simulink library "UAS_Model_library"  (R2018b)
settings: Solver=VariableStepAuto  StartTime=0.0  StopTime=10.0  RelTol=1e-3
undefined symbols (not defined in the file): B, CBAR, CD_alpha, CL_alpha, Cl_beta, Cl_del_a, CL_del_e, Cl_del_r, Cl_p, CL_q, Cl_r, CL_u, Cm_alpha, Cm_alpha_dot, Cm_del_e, Cm_q, Cm_u, Cn_beta, Cn_del_a, Cn_del_r, Cn_p, Cn_r, CY_beta, CY_del_r, CY_p, CY_r, ETA, F, I_TENSOR, Init_Euler, Init_Pos, Init_Rate, Init_Vel, K_p, K_q, K_r, K_roll, K_theta, K_vt, Light, Mass, Max_del_a, Max_del_e, Max_del_r, Max_del_T, MIL, S, tau_a, tau_e, tau_r, tau_T, u_trim, UNIT_GRAV, UNIT_HP2W, XCG, XCGR, XPROP
libraries: aerolibwind2 x3, aerolibasang x3, shared6dofsys x2, aerolibtransform2 x2, aerolibatmos2 x1, sharedtransform x1, sharedutil x1, shared6dof x1, aerolibbdyn x1
settings Model: Creator=e804440  LastModifiedBy=e804440

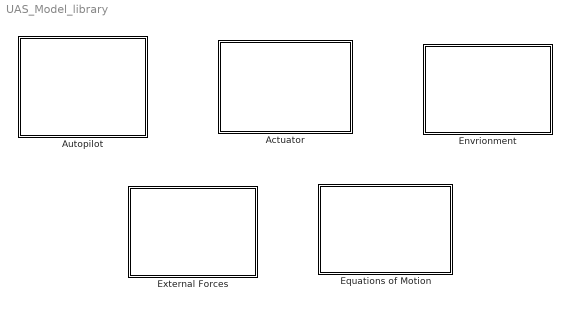
== system UAS_Model_library ==
  Actuator : Subsystem
  Autopilot : Subsystem
  Envrionment : Subsystem
  Equations of Motion : Subsystem
  External Forces : Subsystem

== system UAS_Model_library/Actuator ==
  Aileron Servo : Subsystem
  Elevator Servo : Subsystem
  Rudder Servo : Subsystem
  Throttle Servo : Subsystem

== system UAS_Model_library/Autopilot ==
  Pitch Control : Subsystem
  Roll Control : Subsystem
  Speed Control : Subsystem
  Yaw SAS : Subsystem

== system UAS_Model_library/Envrionment ==
  Atmosphere Model : Subsystem
  Gravity : Subsystem
  Wind Model : Subsystem

== system UAS_Model_library/Equations of Motion ==
  Altitude : Subsystem
  Calculate DCM & Euler Angles : Subsystem
  Calculate omega_dot : shared6dofsys/Calculate omega_dot  aMode=aMode
      settings: SourceProductName=Aerospace Blockset  SourceProductBaseCode=AE
  "Determine Force, Moment & Inertia" : Subsystem
  Vbxw : sharedutil/3x3 Cross Product  aMode=aMode
      settings: SourceProductBaseCode=AE
  "p,q,r " : Integrator  InitialCondition=Init_Rate
  "transform to Inertial axes " : shared6dof/6DOF (Euler Angles)/transform to Inertial axes   SystemSampleTime=-1
      settings: SourceProductName=Aerospace Blockset  SourceProductBaseCode=AE
  ub,vb,wb : Integrator  InitialCondition=Init_Vel
  xe,ye,ze : Integrator  InitialCondition=Init_Pos

== system UAS_Model_library/External Forces ==
  Aerodynamics : Subsystem
  Propulsive : Subsystem
  Total Force & Moment : Subsystem

== system UAS_Model_library/Actuator/Aileron Servo ==
  del_a_cmd : Inport
  Aileron Limit : Saturate  UpperLimit=Max_del_a  LowerLimit=-Max_del_a
  Aileron Servo : TransferFcn  Denominator=[tau_a 1]
  Sum2 : Sum  SaturateOnIntegerOverflow=on
  Trim del_T2 : Constant  Value=u_trim(3)
  del_a : Outport
  wires:
  Trim del_T2/1 -> Sum2/2
  Sum2/1 -> Aileron Limit/1
  del_a_cmd/1 -> Aileron Servo/1
  Aileron Servo/1 -> Sum2/1
  Aileron Limit/1 -> del_a/1

== system UAS_Model_library/Actuator/Elevator Servo ==
  del_e_cmd : Inport
  Elevator Limit : Saturate  UpperLimit=Max_del_e  LowerLimit=-Max_del_e
  Elevator Servo : TransferFcn  Numerator=[-1]  Denominator=[tau_e 1]
  Sum1 : Sum  SaturateOnIntegerOverflow=on
  Trim del_T1 : Constant  Value=u_trim(2)
  del_e : Outport
  wires:
  Sum1/1 -> Elevator Limit/1
  del_e_cmd/1 -> Elevator Servo/1
  Trim del_T1/1 -> Sum1/2
  Elevator Servo/1 -> Sum1/1
  Elevator Limit/1 -> del_e/1

== system UAS_Model_library/Actuator/Rudder Servo ==
  del_r_cmd : Inport
  Rudder Limit : Saturate  UpperLimit=Max_del_r  LowerLimit=-Max_del_r
  Rudder Servo : TransferFcn  Numerator=[-1]  Denominator=[tau_r 1]
  Sum3 : Sum  SaturateOnIntegerOverflow=on
  Trim del_T3 : Constant  Value=u_trim(4)
  del_r : Outport
  wires:
  Trim del_T3/1 -> Sum3/2
  Rudder Limit/1 -> del_r/1
  Rudder Servo/1 -> Sum3/1
  del_r_cmd/1 -> Rudder Servo/1
  Sum3/1 -> Rudder Limit/1

== system UAS_Model_library/Actuator/Throttle Servo ==
  del_T_cmd : Inport
  Sum : Sum  SaturateOnIntegerOverflow=on
  Throttle Limit : Saturate  UpperLimit=Max_del_T  LowerLimit=-Max_del_T
  Throttle Servo : TransferFcn  Denominator=[tau_T 1]
  Trim del_T : Constant  Value=u_trim(1)
  del_T : Outport
  wires:
  del_T_cmd/1 -> Throttle Servo/1
  Sum/1 -> Throttle Limit/1
  Throttle Servo/1 -> Sum/1
  Trim del_T/1 -> Sum/2
  Throttle Limit/1 -> del_T/1

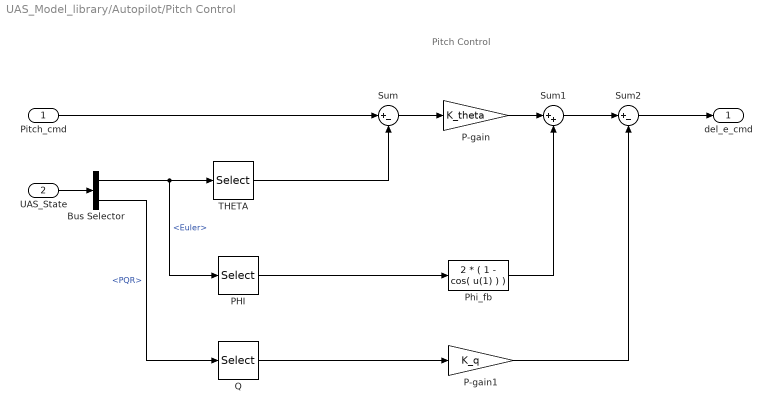
== system UAS_Model_library/Autopilot/Pitch Control ==
  note: Pitch Control
  Pitch_cmd : Inport
  UAS_State : Inport  Port=2
  Bus Selector : BusSelector  OutputSignals=Euler,PQR
  P-gain : Gain  Gain=K_theta
  P-gain1 : Gain  Gain=K_q
  PHI : Selector  InputPortWidth=3  IndexOptions=Index vector (dialog)  Indices=[1]  OutputSizes=1
  Phi_fb : Fcn  Expr=2 * ( 1 - cos( u(1) ) )
  Q : Selector  InputPortWidth=3  IndexOptions=Index vector (dialog)  Indices=[2]  OutputSizes=1
  Sum : Sum  Inputs=|+-
  Sum1 : Sum  Inputs=|++
  Sum2 : Sum  Inputs=|+-
  THETA : Selector  InputPortWidth=3  IndexOptions=Index vector (dialog)  Indices=[2]  OutputSizes=1
  del_e_cmd : Outport
  wires:
  Pitch_cmd/1 -> Sum/1
  Sum/1 -> P-gain/1
  THETA/1 -> Sum/2
  P-gain/1 -> Sum1/1
  Q/1 -> P-gain1/1
  PHI/1 -> Phi_fb/1
  Phi_fb/1 -> Sum1/2
  Sum1/1 -> Sum2/1
  P-gain1/1 -> Sum2/2
  Sum2/1 -> del_e_cmd/1
  Bus Selector/1 -> PHI/1, THETA/1  "<Euler>"
  UAS_State/1 -> Bus Selector/1
  Bus Selector/2 -> Q/1  "<PQR>"

== system UAS_Model_library/Autopilot/Roll Control ==
  note: Roll Control
  Roll_cmd : Inport
  UAS_State : Inport  Port=2
  Bus Selector : BusSelector  OutputSignals=Euler,PQR
  Discrete Transfer Fcn : DiscreteTransferFcn  Numerator=[K_roll -K_roll]  Denominator=[1 -1]
  P : Selector  InputPortWidth=3  IndexOptions=Index vector (dialog)  Indices=[1]  OutputSizes=1
  P-gain1 : Gain  Gain=K_p
  PHI : Selector  InputPortWidth=3  IndexOptions=Index vector (dialog)  Indices=[1]  OutputSizes=1
  Sum : Sum  Inputs=|+-
  Sum2 : Sum  Inputs=|+-
  del_a_cmd : Outport
  wires:
  Sum2/1 -> del_a_cmd/1
  P-gain1/1 -> Sum2/2
  Discrete Transfer Fcn/1 -> Sum2/1
  P/1 -> P-gain1/1
  Sum/1 -> Discrete Transfer Fcn/1
  Roll_cmd/1 -> Sum/1
  PHI/1 -> Sum/2
  UAS_State/1 -> Bus Selector/1
  Bus Selector/1 -> PHI/1  "<Euler>"
  Bus Selector/2 -> P/1  "<PQR>"

== system UAS_Model_library/Autopilot/Speed Control ==
  note: Speed Control
  Speed_cmd : Inport
  UAS_State : Inport  Port=2
  Bus Selector : BusSelector  OutputSignals=Alpha_Beta_V
  P-gain : Gain  Gain=K_vt
  Sum : Sum  Inputs=|+-
  VT : Selector  InputPortWidth=3  IndexOptions=Index vector (dialog)  Indices=[3]  OutputSizes=1
  del_T_cmd : Outport
  wires:
  P-gain/1 -> del_T_cmd/1
  UAS_State/1 -> Bus Selector/1
  VT/1 -> Sum/2
  Sum/1 -> P-gain/1
  Speed_cmd/1 -> Sum/1
  Bus Selector/1 -> VT/1  "<Alpha_Beta_V>"

== system UAS_Model_library/Autopilot/Yaw SAS ==
  note: Yaw SAS (Stability Augmented System)
  UAS_State : Inport
  Bus Selector : BusSelector  OutputSignals=PQR
  P-gain1 : Gain  Gain=K_r
  R : Selector  InputPortWidth=3  IndexOptions=Index vector (dialog)  Indices=[3]  OutputSizes=1
  del_r_cmd : Outport
  wires:
  UAS_State/1 -> Bus Selector/1
  R/1 -> P-gain1/1
  P-gain1/1 -> del_r_cmd/1
  Bus Selector/1 -> R/1  "<PQR>"

== system UAS_Model_library/Envrionment/Atmosphere Model ==
  Alt : Inport
  ISA Atmosphere Model : aerolibatmos2/ISA Atmosphere Model  custom=off  g=9.80665  gamma=1.4  R=287.0531  L=0.0065  h_trop=11000  h_strat=20000  rho0=1.225  P0=101325  T0=288.15  h0=0
      settings: SourceProductName=Aerospace Blockset
  Terminator : Terminator
  Terminator1 : Terminator
  a : Outport
  rho : Outport  Port=2
  wires:
  ISA Atmosphere Model/3 -> Terminator1/1
  ISA Atmosphere Model/1 -> Terminator/1
  ISA Atmosphere Model/4 -> rho/1
  Alt/1 -> ISA Atmosphere Model/1
  ISA Atmosphere Model/2 -> a/1

== system UAS_Model_library/Envrionment/Gravity ==
  cE_B : Inport
  Constant : Constant  Value=0
  Constant1 : Constant  Value=Mass
  "Gravity vector in body frame " : Product  Multiplication=Matrix(*)  SaturateOnIntegerOverflow=on  InputSameDT=on  OutDataTypeStr=Inherit: Same as first input
  Mux1 : Mux  Inputs=3
  g : Gain  Gain=UNIT_GRAV
  Gravity : Outport
  wires:
  Constant/1 -> Mux1/2, Mux1/1
  cE_B/1 -> "Gravity vector in body frame "/1
  Mux1/1 -> "Gravity vector in body frame "/2
  g/1 -> Mux1/3
  "Gravity vector in body frame "/1 -> Gravity/1
  Constant1/1 -> g/1

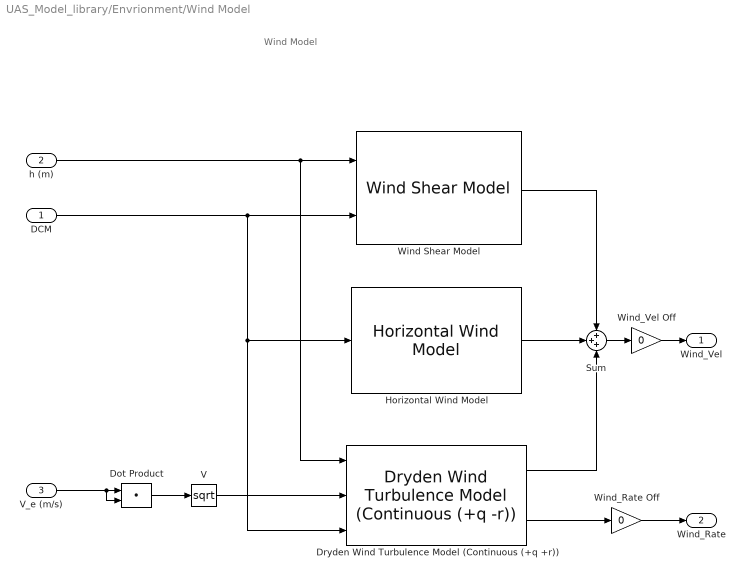
== system UAS_Model_library/Envrionment/Wind Model ==
  note: Wind Model
  DCM : Inport
  h (m) : Inport  Port=2
  V_e (m/s) : Inport  Port=3
  Dot Product : DotProduct  SaturateOnIntegerOverflow=on  OutDataTypeStr=Inherit: Inherit via internal rule
  Dryden Wind Turbulence Model (Continuous (+q +r)) : aerolibwind2/Dryden Wind Turbulence Model  (Continuous (+q -r))  units=Metric (MKS)  spec=MIL-F-8785C  model=Continuous Dryden (+q -r)  W20=15  Wdeg=0  TurbProb=10^-2 - Light  L_high=533.4  Wingspan=B  ts=Step_Size  Seed=[23341 23342 23343 23344]  T_on=off
      settings: SourceProductName=Aerospace Blockset
  Horizontal Wind Model : aerolibwind2/Horizontal Wind Model  units=Metric (MKS)  Vw_source=Internal  Vwind=0  W_source=Internal  Wdeg=0
      settings: SourceProductName=Aerospace Blockset  SourceProductBaseCode=AE
  Sum : Sum  Inputs=+++  SaturateOnIntegerOverflow=on  InputSameDT=on  OutDataTypeStr=Inherit: Same as first input
  V : Math  Operator=sqrt  SaturateOnIntegerOverflow=on
  Wind Shear Model : aerolibwind2/Wind Shear Model  units=Metric (MKS)  phase=Category C - Terminal Flight Phase  W_20=0  Wdeg=0
      settings: SourceProductName=Aerospace Blockset
  Wind_Rate Off : Gain  Gain=0
  Wind_Vel Off : Gain  Gain=0
  Wind_Vel : Outport
  Wind_Rate : Outport  Port=2
  wires:
  Wind_Rate Off/1 -> Wind_Rate/1
  Wind_Vel Off/1 -> Wind_Vel/1
  V/1 -> Dryden Wind Turbulence Model (Continuous (+q +r))/2
  DCM/1 -> Wind Shear Model/2, Horizontal Wind Model/1, Dryden Wind Turbulence Model (Continuous (+q +r))/3
  h (m)/1 -> Wind Shear Model/1, Dryden Wind Turbulence Model (Continuous (+q +r))/1
  Dryden Wind Turbulence Model (Continuous (+q +r))/1 -> Sum/3
  V_e (m/s)/1 -> Dot Product/1, Dot Product/2
  Dot Product/1 -> V/1
  Dryden Wind Turbulence Model (Continuous (+q +r))/2 -> Wind_Rate Off/1
  Sum/1 -> Wind_Vel Off/1
  Horizontal Wind Model/1 -> Sum/2
  Wind Shear Model/1 -> Sum/1

== system UAS_Model_library/Equations of Motion/Altitude ==
  Xe : Inport
  Z_e : Selector  InputPortWidth=3  IndexOptions=Index vector (dialog)  Indices=[3]  OutputSizes=1
  conv : Gain  Gain=-1
  h : Outport
  wires:
  conv/1 -> h/1
  Z_e/1 -> conv/1
  Xe/1 -> Z_e/1

== system UAS_Model_library/Equations of Motion/Calculate DCM & Euler Angles ==
  "p q r " : Inport
  Rotation Angles to Direction Cosine Matrix : sharedtransform/Rotation Angles to Direction Cosine Matrix  rotationOrder=ZYX  aMode=aMode
      settings: SourceProductBaseCode=AE
  Selector : Selector  InputPortWidth=3  IndexOptions=Index vector (dialog)  Indices=[3 2 1]  OutputSizes=1
  phi theta psi : Integrator  InitialCondition=Init_Euler
  phidot thetadot psidot : shared6dofsys/DCM & Euler Angles (Euler)/phidot thetadot psidot  SystemSampleTime=-1
      settings: SourceProductName=Aerospace Blockset  SourceProductBaseCode=AE
  DCM : Outport
  Euler : Outport  Port=2
  wires:
  Selector/1 -> Rotation Angles to Direction Cosine Matrix/1
  phi theta psi/1 -> phidot thetadot psidot/2, Selector/1, Euler/1
  phidot thetadot psidot/1 -> phi theta psi/1
  "p q r "/1 -> phidot thetadot psidot/1
  Rotation Angles to Direction Cosine Matrix/1 -> DCM/1

== system UAS_Model_library/Equations of Motion/Determine Force, Moment & Inertia ==
  forces : Inport
  Constant : Constant  Value=Mass  OutDataTypeStr=Inherit: Inherit via back propagation
  Constant1 : Constant  Value=I_TENSOR  OutDataTypeStr=Inherit: Inherit via back propagation
  Constant2 : Constant  Value=zeros(3)
  Vector Concatenate : Concatenate  Mode=Multidimensional array
  "forces " : Outport
  mass : Outport  Port=2
  "inertia, 0" : Outport  Port=3
  wires:
  Vector Concatenate/1 -> "inertia, 0"/1
  Constant2/1 -> Vector Concatenate/2
  Constant1/1 -> Vector Concatenate/1
  forces/1 -> "forces "/1
  Constant/1 -> mass/1

== system UAS_Model_library/External Forces/Aerodynamics ==
  Aerodynamic Force & Moment : Subsystem
  Aerodynamics coefficients : Subsystem
  Direction Cosine Matrix Body to Wind : aerolibtransform2/Direction Cosine Matrix Body to Wind
      settings: SourceProductName=Aerospace Blockset  SourceProductBaseCode=AE
  Wind-axes Velocitie : Subsystem

== system UAS_Model_library/External Forces/Propulsive ==
  Propulsive Force & Moment : Subsystem

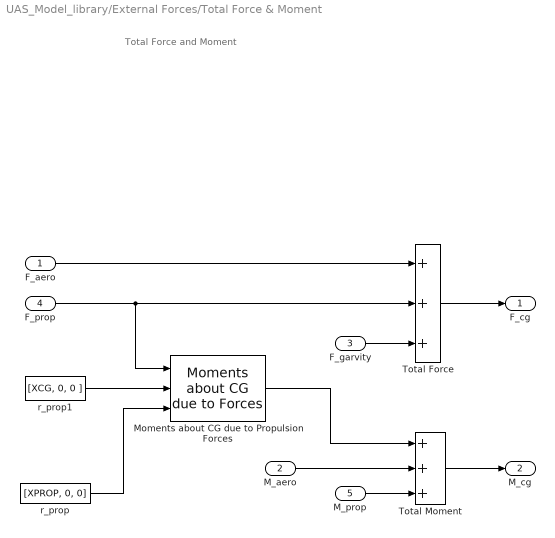
== system UAS_Model_library/External Forces/Total Force & Moment ==
  note: Total Force and Moment
  F_aero : Inport  PortDimensions=3
  M_aero : Inport  Port=2  PortDimensions=3
  F_garvity : Inport  Port=3  PortDimensions=3
  F_prop : Inport  Port=4  PortDimensions=3
  M_prop : Inport  Port=5  PortDimensions=3
  Moments about CG due to Propulsion Forces : aerolibbdyn/Moments about CG  due to Forces
      settings: SourceProductName=Aerospace Blockset  SourceProductBaseCode=AE
  Total Force : Sum  Inputs=+++  SaturateOnIntegerOverflow=on  InputSameDT=on  OutDataTypeStr=Inherit: Same as first input
  Total Moment : Sum  Inputs=+++  SaturateOnIntegerOverflow=on  InputSameDT=on  OutDataTypeStr=Inherit: Same as first input
  r_prop : Constant  Value=[XPROP, 0, 0]  OutDataTypeStr=double
  r_prop1 : Constant  Value=[XCG, 0, 0 ]  OutDataTypeStr=double
  F_cg : Outport
  M_cg : Outport  Port=2
  wires:
  M_aero/1 -> Total Moment/2
  Moments about CG due to Propulsion Forces/1 -> Total Moment/1
  Total Force/1 -> F_cg/1
  F_aero/1 -> Total Force/1
  F_prop/1 -> Moments about CG due to Propulsion Forces/1, Total Force/2
  M_prop/1 -> Total Moment/3
  Total Moment/1 -> M_cg/1
  r_prop/1 -> Moments about CG due to Propulsion Forces/3
  r_prop1/1 -> Moments about CG due to Propulsion Forces/2
  F_garvity/1 -> Total Force/3

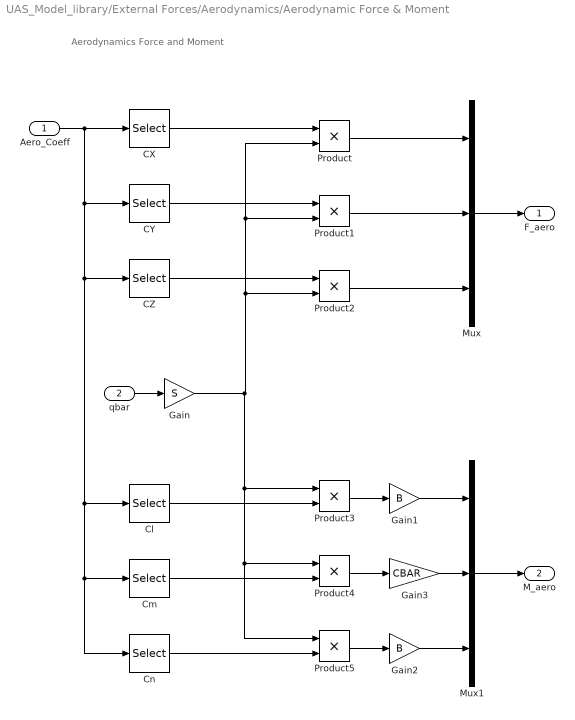
== system UAS_Model_library/External Forces/Aerodynamics/Aerodynamic Force & Moment ==
  note: Aerodynamics Force and Moment
  Aero_Coeff : Inport
  qbar : Inport  Port=2
  CX : Selector  InputPortWidth=6  IndexOptions=Index vector (dialog)  Indices=[1]  OutputSizes=1
  CY : Selector  InputPortWidth=6  IndexOptions=Index vector (dialog)  Indices=[2]  OutputSizes=1
  CZ : Selector  InputPortWidth=6  IndexOptions=Index vector (dialog)  Indices=[3]  OutputSizes=1
  Cl : Selector  InputPortWidth=6  IndexOptions=Index vector (dialog)  Indices=[4]  OutputSizes=1
  Cm : Selector  InputPortWidth=6  IndexOptions=Index vector (dialog)  Indices=[5]  OutputSizes=1
  Cn : Selector  InputPortWidth=6  IndexOptions=Index vector (dialog)  Indices=[6]  OutputSizes=1
  Gain : Gain  Gain=S
  Gain1 : Gain  Gain=B
  Gain2 : Gain  Gain=B
  Gain3 : Gain  Gain=CBAR
  Mux : Mux  Inputs=3
  Mux1 : Mux  Inputs=3
  Product{,1..5} (6 alike) : Product
  F_aero : Outport
  M_aero : Outport  Port=2
  wires:
  Aero_Coeff/1 -> Cl/1, Cn/1, Cm/1, CZ/1, CY/1, CX/1
  qbar/1 -> Gain/1
  CX/1 -> Product/1
  Gain/1 -> Product5/1, Product4/1, Product3/1, Product2/2, Product1/2, Product/2
  CY/1 -> Product1/1
  CZ/1 -> Product2/1
  Product/1 -> Mux/1
  Product1/1 -> Mux/2
  Product2/1 -> Mux/3
  Mux/1 -> F_aero/1
  Cl/1 -> Product3/2
  Cm/1 -> Product4/2
  Cn/1 -> Product5/2
  Product3/1 -> Gain1/1
  Product4/1 -> Gain3/1
  Product5/1 -> Gain2/1
  Mux1/1 -> M_aero/1
  Gain1/1 -> Mux1/1
  Gain2/1 -> Mux1/3
  Gain3/1 -> Mux1/2

== system UAS_Model_library/External Forces/Aerodynamics/Aerodynamics coefficients ==
  Drag Force Coefficient : Subsystem
  "Lift Force Coefficient  " : Subsystem
  Pitching Moment Coefficient : Subsystem
  Rolling Moment Coefficient : Subsystem
  "Side Force Coefficient " : Subsystem
  Yawing Moment Coefficient : Subsystem

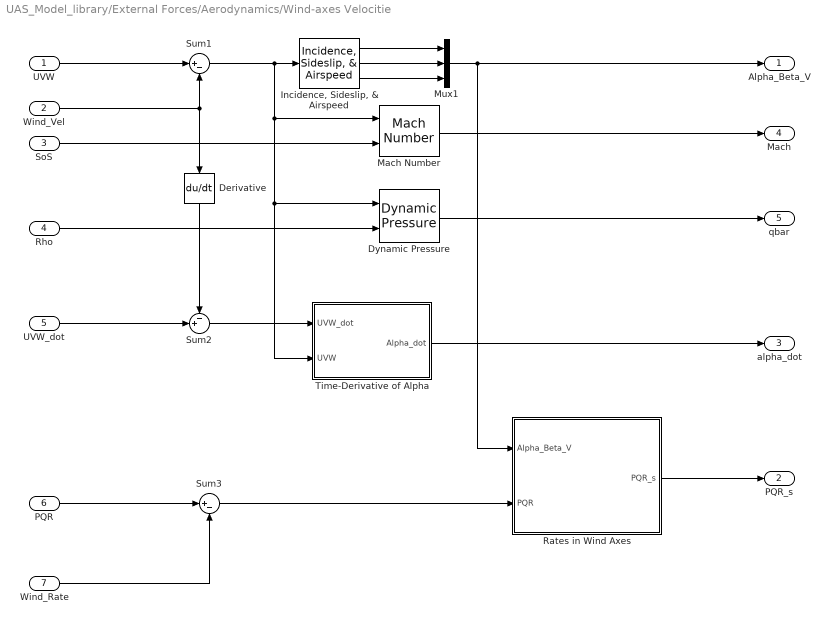
== system UAS_Model_library/External Forces/Aerodynamics/Wind-axes Velocitie ==
  UVW : Inport
  Wind_Vel : Inport  Port=2
  SoS : Inport  Port=3
  Rho : Inport  Port=4
  UVW_dot : Inport  Port=5
  PQR : Inport  Port=6
  Wind_Rate : Inport  Port=7
  Derivative : Derivative
  Dynamic Pressure : aerolibasang/Dynamic Pressure
  "Incidence, Sideslip, & Airspeed" : aerolibasang/Incidence, Sideslip, & Airspeed
      settings: SourceProductName=Aerospace Blockset
  Mach Number : aerolibasang/Mach Number
      settings: SourceProductName=Aerospace Blockset  SourceProductBaseCode=AE
  Mux1 : Mux  Inputs=3
  Rates in Wind Axes : Subsystem
  Sum1 : Sum  Inputs=|+-  SaturateOnIntegerOverflow=on  InputSameDT=on  OutDataTypeStr=Inherit: Same as first input
  Sum2 : Sum  Inputs=-+|  SaturateOnIntegerOverflow=on  InputSameDT=on  OutDataTypeStr=Inherit: Same as first input
  Sum3 : Sum  Inputs=|+-  SaturateOnIntegerOverflow=on  InputSameDT=on  OutDataTypeStr=Inherit: Same as first input
  Time-Derivative of Alpha : Subsystem
  Alpha_Beta_V : Outport
  PQR_s : Outport  Port=2
  alpha_dot : Outport  Port=3
  Mach : Outport  Port=4
  qbar : Outport  Port=5
  wires:
  Derivative/1 -> Sum2/1
  Sum2/1 -> Time-Derivative of Alpha/1(UVW_dot)
  UVW_dot/1 -> Sum2/2
  Time-Derivative of Alpha/1(Alpha_dot) -> alpha_dot/1
  Dynamic Pressure/1 -> qbar/1
  Rho/1 -> Dynamic Pressure/2
  SoS/1 -> Mach Number/2
  Mach Number/1 -> Mach/1
  Wind_Vel/1 -> Sum1/2, Derivative/1
  UVW/1 -> Sum1/1
  Mux1/1 -> Rates in Wind Axes/1(Alpha_Beta_V), Alpha_Beta_V/1
  Sum1/1 -> Time-Derivative of Alpha/2(UVW), Dynamic Pressure/1, Mach Number/1, "Incidence, Sideslip, & Airspeed"/1
  "Incidence, Sideslip, & Airspeed"/1 -> Mux1/1
  "Incidence, Sideslip, & Airspeed"/2 -> Mux1/2
  "Incidence, Sideslip, & Airspeed"/3 -> Mux1/3
  Rates in Wind Axes/1(PQR_s) -> PQR_s/1
  Sum3/1 -> Rates in Wind Axes/2(PQR)
  PQR/1 -> Sum3/1
  Wind_Rate/1 -> Sum3/2

== system UAS_Model_library/External Forces/Propulsive/Propulsive Force & Moment ==
  note: Propulsive Force and Moment
  Controls : Inport
  Alpha_Beta_V : Inport  Port=2
  Constant : Constant  Value=0
  Engine Thrust : Product  Inputs=*/
  Gain : Gain  Gain=ETA
  Gain1 : Gain  Gain=UNIT_HP2W
  Mux : Mux  Inputs=3
  Mux1 : Mux  Inputs=3
  V : Selector  InputPortWidth=3  IndexOptions=Index vector (dialog)  Indices=[3]  OutputSizes=1
  del_T (HP) : Selector  InputPortWidth=4  IndexOptions=Index vector (dialog)  Indices=[1]  OutputSizes=1
  F_prop : Outport
  M_prop : Outport  Port=2
  wires:
  Mux1/1 -> M_prop/1
  Constant/1 -> Mux/3, Mux1/3, Mux1/2, Mux1/1, Mux/2
  Controls/1 -> del_T (HP)/1
  del_T (HP)/1 -> Gain1/1
  Gain1/1 -> Gain/1
  Gain/1 -> Engine Thrust/1  "Engine Power"
  Engine Thrust/1 -> Mux/1
  Alpha_Beta_V/1 -> V/1
  V/1 -> Engine Thrust/2
  Mux/1 -> F_prop/1

== system UAS_Model_library/External Forces/Aerodynamics/Aerodynamics coefficients/Drag Force Coefficient ==
  note: Drag Force Coefficient
  Alpha_Beta_V : Inport
  Alpha : Selector  InputPortWidth=3  IndexOptions=Index vector (dialog)  Indices=[1]  OutputSizes=1
  Gain : Gain  Gain=CD_alpha
  CD : Outport
  wires:
  Alpha_Beta_V/1 -> Alpha/1
  Alpha/1 -> Gain/1
  Gain/1 -> CD/1

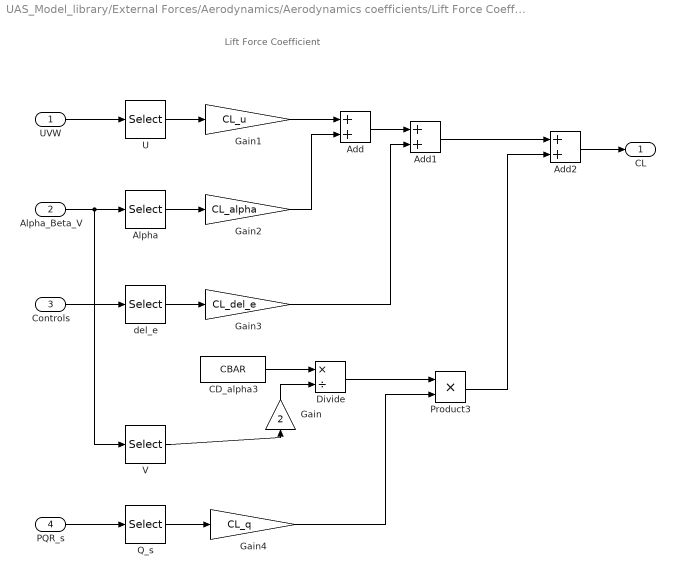
== system UAS_Model_library/External Forces/Aerodynamics/Aerodynamics coefficients/Lift Force Coefficient   ==
  note: Lift Force Coefficient
  UVW : Inport
  Alpha_Beta_V : Inport  Port=2
  Controls : Inport  Port=3
  PQR_s : Inport  Port=4
  Add : Sum
  Add1 : Sum
  Add2 : Sum
  Alpha : Selector  InputPortWidth=3  IndexOptions=Index vector (dialog)  Indices=[1]  OutputSizes=1
  CD_alpha3 : Constant  Value=CBAR
  Divide : Product  Inputs=*/
  Gain : Gain  Gain=2
  Gain1 : Gain  Gain=CL_u
  Gain2 : Gain  Gain=CL_alpha
  Gain3 : Gain  Gain=CL_del_e
  Gain4 : Gain  Gain=CL_q
  Product3 : Product
  Q_s : Selector  InputPortWidth=3  IndexOptions=Index vector (dialog)  Indices=[2]  OutputSizes=1
  U : Selector  InputPortWidth=3  IndexOptions=Index vector (dialog)  Indices=[1]  OutputSizes=1
  V : Selector  InputPortWidth=3  IndexOptions=Index vector (dialog)  Indices=[3]  OutputSizes=1
  del_e : Selector  InputPortWidth=4  IndexOptions=Index vector (dialog)  Indices=[2]  OutputSizes=1
  CL : Outport
  wires:
  UVW/1 -> U/1
  Alpha_Beta_V/1 -> Alpha/1, V/1
  Gain2/1 -> Add/2
  Controls/1 -> del_e/1
  Add/1 -> Add1/1
  Gain3/1 -> Add1/2
  CD_alpha3/1 -> Divide/1
  Gain/1 -> Divide/2
  Divide/1 -> Product3/1
  Add1/1 -> Add2/1
  Product3/1 -> Add2/2
  Add2/1 -> CL/1
  Gain4/1 -> Product3/2
  PQR_s/1 -> Q_s/1
  U/1 -> Gain1/1
  Alpha/1 -> Gain2/1
  del_e/1 -> Gain3/1
  V/1 -> Gain/1
  Q_s/1 -> Gain4/1
  Gain1/1 -> Add/1

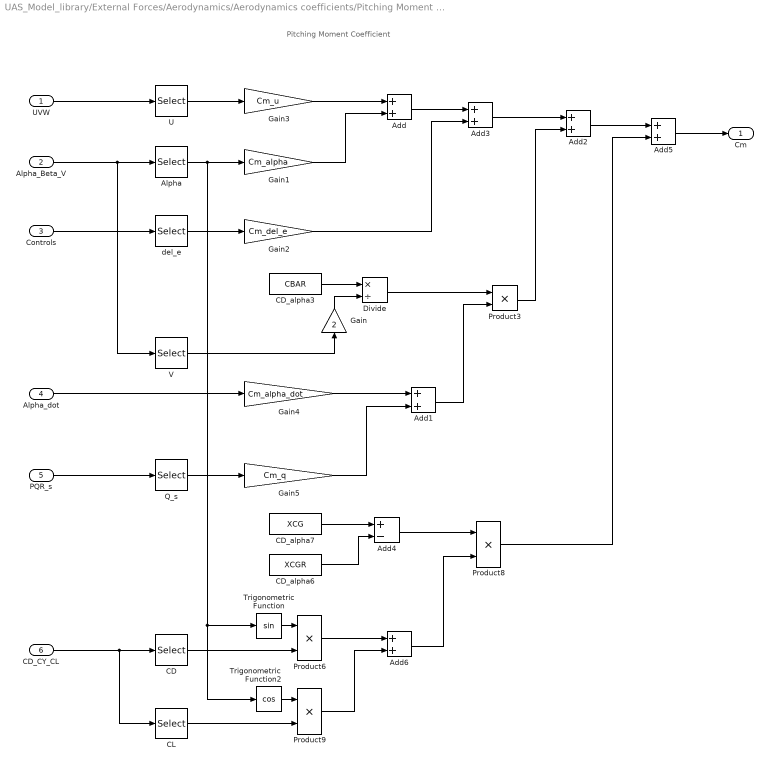
== system UAS_Model_library/External Forces/Aerodynamics/Aerodynamics coefficients/Pitching Moment Coefficient ==
  note: Pitching Moment Coefficient
  UVW : Inport
  Alpha_Beta_V : Inport  Port=2
  Controls : Inport  Port=3
  Alpha_dot : Inport  Port=4
  PQR_s : Inport  Port=5
  CD_CY_CL : Inport  Port=6
  Add{,1..3,5..6} (6 alike) : Sum
  Add4 : Sum  Inputs=+-
  Alpha : Selector  InputPortWidth=3  IndexOptions=Index vector (dialog)  Indices=[1]  OutputSizes=1
  CD : Selector  InputPortWidth=3  IndexOptions=Index vector (dialog)  Indices=[1]  OutputSizes=1
  CD_alpha3 : Constant  Value=CBAR
  CD_alpha6 : Constant  Value=XCGR
  CD_alpha7 : Constant  Value=XCG
  CL : Selector  InputPortWidth=3  IndexOptions=Index vector (dialog)  Indices=[3]  OutputSizes=1
  Divide : Product  Inputs=*/
  Gain : Gain  Gain=2
  Gain1 : Gain  Gain=Cm_alpha
  Gain2 : Gain  Gain=Cm_del_e
  Gain3 : Gain  Gain=Cm_u
  Gain4 : Gain  Gain=Cm_alpha_dot
  Gain5 : Gain  Gain=Cm_q
  Product{3,6,8..9} (4 alike) : Product
  Q_s : Selector  InputPortWidth=3  IndexOptions=Index vector (dialog)  Indices=[2]  OutputSizes=1
  Trigonometric Function : Trigonometry
  Trigonometric Function2 : Trigonometry  Operator=cos
  U : Selector  InputPortWidth=3  IndexOptions=Index vector (dialog)  Indices=[1]  OutputSizes=1
  V : Selector  InputPortWidth=3  IndexOptions=Index vector (dialog)  Indices=[3]  OutputSizes=1
  del_e : Selector  InputPortWidth=4  IndexOptions=Index vector (dialog)  Indices=[2]  OutputSizes=1
  Cm : Outport
  wires:
  UVW/1 -> U/1
  Gain3/1 -> Add/1
  Alpha_Beta_V/1 -> V/1, Alpha/1
  Gain1/1 -> Add/2
  CD_alpha3/1 -> Divide/1
  Gain/1 -> Divide/2
  Divide/1 -> Product3/1
  Add/1 -> Add3/1
  Alpha_dot/1 -> Gain4/1
  PQR_s/1 -> Q_s/1
  Product3/1 -> Add2/2
  Controls/1 -> del_e/1
  Gain2/1 -> Add3/2
  Add3/1 -> Add2/1
  CD_CY_CL/1 -> CL/1, CD/1
  Trigonometric Function/1 -> Product6/1
  CD_alpha7/1 -> Add4/1
  CD_alpha6/1 -> Add4/2
  Add4/1 -> Product8/1
  Product8/1 -> Add5/2
  Add2/1 -> Add5/1
  Add5/1 -> Cm/1
  Gain5/1 -> Add1/2
  Add1/1 -> Product3/2
  Product6/1 -> Add6/1
  Trigonometric Function2/1 -> Product9/1
  Product9/1 -> Add6/2
  Add6/1 -> Product8/2
  U/1 -> Gain3/1
  Alpha/1 -> Gain1/1, Trigonometric Function/1, Trigonometric Function2/1
  del_e/1 -> Gain2/1
  V/1 -> Gain/1
  Q_s/1 -> Gain5/1
  CD/1 -> Product6/2
  CL/1 -> Product9/2
  Gain4/1 -> Add1/1

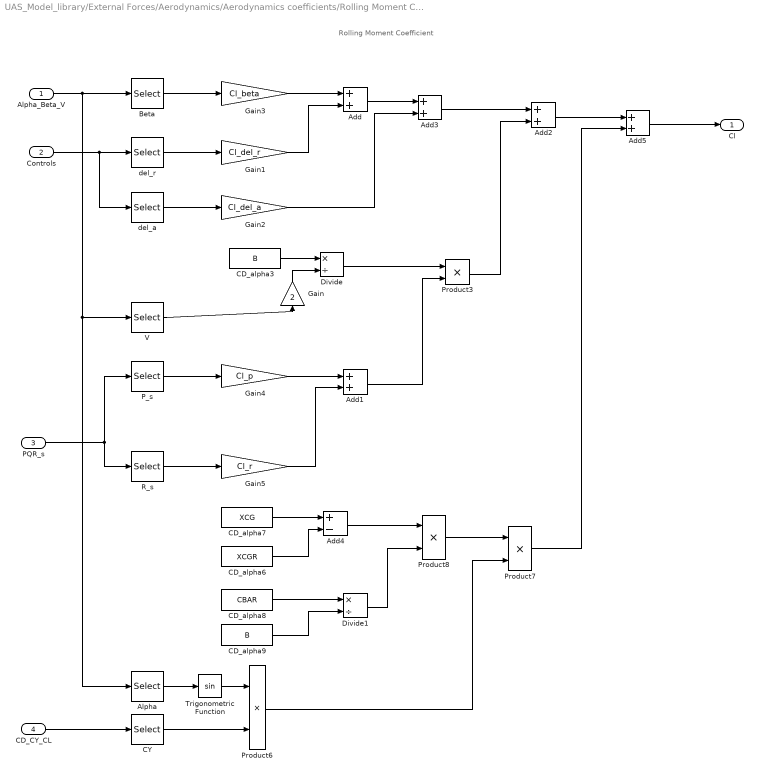
== system UAS_Model_library/External Forces/Aerodynamics/Aerodynamics coefficients/Rolling Moment Coefficient ==
  note: Rolling Moment Coefficient
  Alpha_Beta_V : Inport
  Controls : Inport  Port=2
  PQR_s : Inport  Port=3
  CD_CY_CL : Inport  Port=4
  Add{,1..3,5} (5 alike) : Sum
  Add4 : Sum  Inputs=+-
  Alpha : Selector  InputPortWidth=3  IndexOptions=Index vector (dialog)  Indices=[1]  OutputSizes=1
  Beta : Selector  InputPortWidth=3  IndexOptions=Index vector (dialog)  Indices=[2]  OutputSizes=1
  CD_alpha3 : Constant  Value=B
  CD_alpha6 : Constant  Value=XCGR
  CD_alpha7 : Constant  Value=XCG
  CD_alpha8 : Constant  Value=CBAR
  CD_alpha9 : Constant  Value=B
  CY : Selector  InputPortWidth=3  IndexOptions=Index vector (dialog)  Indices=[2]  OutputSizes=1
  Divide : Product  Inputs=*/
  Divide1 : Product  Inputs=*/
  Gain : Gain  Gain=2
  Gain1 : Gain  Gain=Cl_del_r
  Gain2 : Gain  Gain=Cl_del_a
  Gain3 : Gain  Gain=Cl_beta
  Gain4 : Gain  Gain=Cl_p
  Gain5 : Gain  Gain=Cl_r
  P_s : Selector  InputPortWidth=3  IndexOptions=Index vector (dialog)  Indices=[1]  OutputSizes=1
  Product{3,6..8} (4 alike) : Product
  R_s : Selector  InputPortWidth=3  IndexOptions=Index vector (dialog)  Indices=[3]  OutputSizes=1
  Trigonometric Function : Trigonometry
  V : Selector  InputPortWidth=3  IndexOptions=Index vector (dialog)  Indices=[3]  OutputSizes=1
  del_a : Selector  InputPortWidth=4  IndexOptions=Index vector (dialog)  Indices=[3]  OutputSizes=1
  del_r : Selector  InputPortWidth=4  IndexOptions=Index vector (dialog)  Indices=[4]  OutputSizes=1
  Cl : Outport
  wires:
  Alpha_Beta_V/1 -> Alpha/1, V/1, Beta/1
  Gain3/1 -> Add/1
  Controls/1 -> del_a/1, del_r/1
  Gain1/1 -> Add/2
  CD_alpha3/1 -> Divide/1
  Gain/1 -> Divide/2
  Divide/1 -> Product3/1
  Add/1 -> Add3/1
  Gain4/1 -> Add1/1
  Gain5/1 -> Add1/2
  Add1/1 -> Product3/2
  Product3/1 -> Add2/2
  Add3/1 -> Add2/1
  Trigonometric Function/1 -> Product6/1
  Product6/1 -> Product7/2
  CD_alpha7/1 -> Add4/1
  CD_alpha6/1 -> Add4/2
  Add4/1 -> Product8/1
  Divide1/1 -> Product8/2
  CD_alpha8/1 -> Divide1/1
  CD_alpha9/1 -> Divide1/2
  Product8/1 -> Product7/1
  Add2/1 -> Add5/1
  Add5/1 -> Cl/1
  Product7/1 -> Add5/2
  PQR_s/1 -> P_s/1, R_s/1
  Beta/1 -> Gain3/1
  del_r/1 -> Gain1/1
  del_a/1 -> Gain2/1
  V/1 -> Gain/1
  P_s/1 -> Gain4/1
  R_s/1 -> Gain5/1
  Alpha/1 -> Trigonometric Function/1
  CY/1 -> Product6/2
  CD_CY_CL/1 -> CY/1
  Gain2/1 -> Add3/2

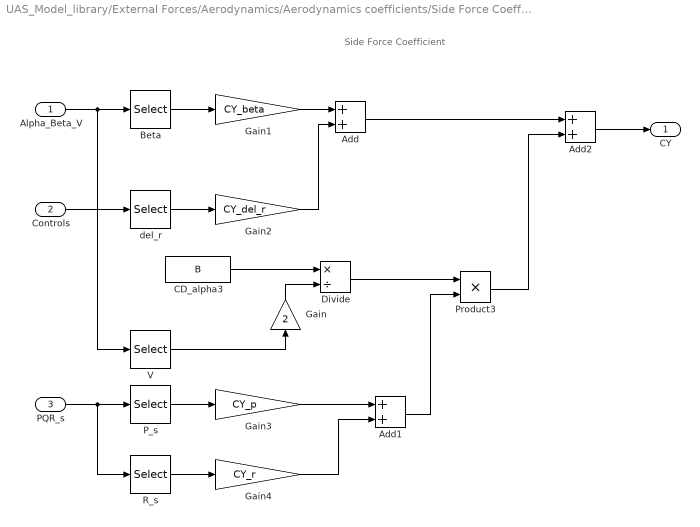
== system UAS_Model_library/External Forces/Aerodynamics/Aerodynamics coefficients/Side Force Coefficient  ==
  note: Side Force Coefficient
  Alpha_Beta_V : Inport
  Controls : Inport  Port=2
  PQR_s : Inport  Port=3
  Add : Sum
  Add1 : Sum
  Add2 : Sum
  Beta : Selector  InputPortWidth=3  IndexOptions=Index vector (dialog)  Indices=[2]  OutputSizes=1
  CD_alpha3 : Constant  Value=B
  Divide : Product  Inputs=*/
  Gain : Gain  Gain=2
  Gain1 : Gain  Gain=CY_beta
  Gain2 : Gain  Gain=CY_del_r
  Gain3 : Gain  Gain=CY_p
  Gain4 : Gain  Gain=CY_r
  P_s : Selector  InputPortWidth=3  IndexOptions=Index vector (dialog)  Indices=[1]  OutputSizes=1
  Product3 : Product
  R_s : Selector  InputPortWidth=3  IndexOptions=Index vector (dialog)  Indices=[3]  OutputSizes=1
  V : Selector  InputPortWidth=3  IndexOptions=Index vector (dialog)  Indices=[3]  OutputSizes=1
  del_r : Selector  InputPortWidth=4  IndexOptions=Index vector (dialog)  Indices=[4]  OutputSizes=1
  CY : Outport
  wires:
  Alpha_Beta_V/1 -> V/1, Beta/1
  Gain1/1 -> Add/1
  Controls/1 -> del_r/1
  CD_alpha3/1 -> Divide/1
  Gain/1 -> Divide/2
  Divide/1 -> Product3/1
  Add/1 -> Add2/1
  Add2/1 -> CY/1
  Add1/1 -> Product3/2
  Product3/1 -> Add2/2
  PQR_s/1 -> R_s/1, P_s/1
  Beta/1 -> Gain1/1
  del_r/1 -> Gain2/1
  V/1 -> Gain/1
  P_s/1 -> Gain3/1
  Gain2/1 -> Add/2
  Gain3/1 -> Add1/1
  R_s/1 -> Gain4/1
  Gain4/1 -> Add1/2

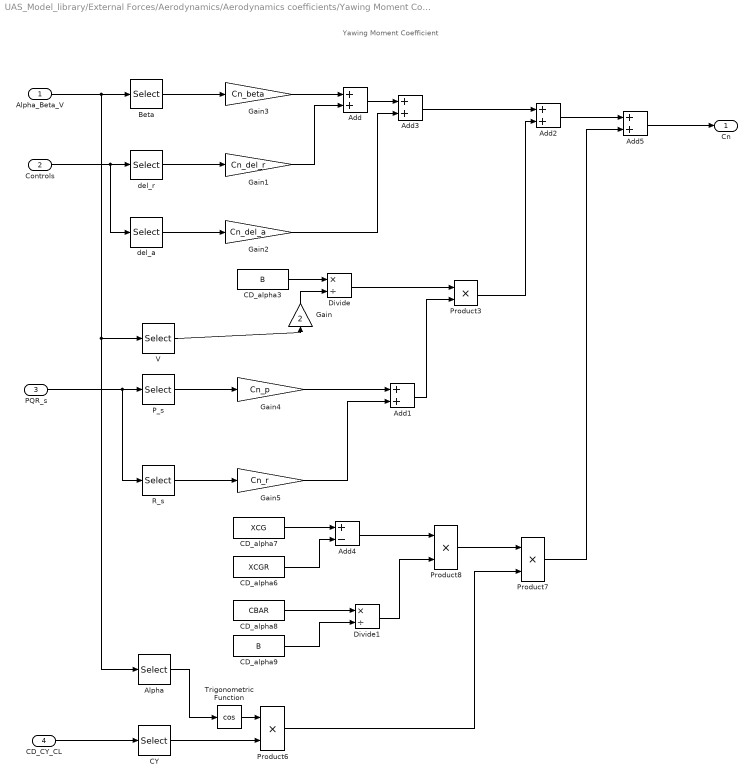
== system UAS_Model_library/External Forces/Aerodynamics/Aerodynamics coefficients/Yawing Moment Coefficient ==
  note: Yawing Moment Coefficient
  Alpha_Beta_V : Inport
  Controls : Inport  Port=2
  PQR_s : Inport  Port=3
  CD_CY_CL : Inport  Port=4
  Add{,1..3,5} (5 alike) : Sum
  Add4 : Sum  Inputs=+-
  Alpha : Selector  InputPortWidth=3  IndexOptions=Index vector (dialog)  Indices=[1]  OutputSizes=1
  Beta : Selector  InputPortWidth=3  IndexOptions=Index vector (dialog)  Indices=[2]  OutputSizes=1
  CD_alpha3 : Constant  Value=B
  CD_alpha6 : Constant  Value=XCGR
  CD_alpha7 : Constant  Value=XCG
  CD_alpha8 : Constant  Value=CBAR
  CD_alpha9 : Constant  Value=B
  CY : Selector  InputPortWidth=3  IndexOptions=Index vector (dialog)  Indices=[2]  OutputSizes=1
  Divide : Product  Inputs=*/
  Divide1 : Product  Inputs=*/
  Gain : Gain  Gain=2
  Gain1 : Gain  Gain=Cn_del_r
  Gain2 : Gain  Gain=Cn_del_a
  Gain3 : Gain  Gain=Cn_beta
  Gain4 : Gain  Gain=Cn_p
  Gain5 : Gain  Gain=Cn_r
  P_s : Selector  InputPortWidth=3  IndexOptions=Index vector (dialog)  Indices=[1]  OutputSizes=1
  Product{3,6..8} (4 alike) : Product
  R_s : Selector  InputPortWidth=3  IndexOptions=Index vector (dialog)  Indices=[3]  OutputSizes=1
  Trigonometric Function : Trigonometry  Operator=cos
  V : Selector  InputPortWidth=3  IndexOptions=Index vector (dialog)  Indices=[3]  OutputSizes=1
  del_a : Selector  InputPortWidth=4  IndexOptions=Index vector (dialog)  Indices=[3]  OutputSizes=1
  del_r : Selector  InputPortWidth=4  IndexOptions=Index vector (dialog)  Indices=[4]  OutputSizes=1
  Cn : Outport
  wires:
  Alpha_Beta_V/1 -> Alpha/1, V/1, Beta/1
  Gain3/1 -> Add/1
  Controls/1 -> del_a/1, del_r/1
  Gain1/1 -> Add/2
  CD_alpha3/1 -> Divide/1
  Gain/1 -> Divide/2
  Divide/1 -> Product3/1
  Add/1 -> Add3/1
  PQR_s/1 -> P_s/1, R_s/1
  Gain4/1 -> Add1/1
  Gain5/1 -> Add1/2
  Add1/1 -> Product3/2
  Product3/1 -> Add2/2
  Add3/1 -> Add2/1
  CD_CY_CL/1 -> CY/1
  Trigonometric Function/1 -> Product6/1
  Product6/1 -> Product7/2
  CD_alpha7/1 -> Add4/1
  CD_alpha6/1 -> Add4/2
  Add4/1 -> Product8/1
  Divide1/1 -> Product8/2
  CD_alpha8/1 -> Divide1/1
  CD_alpha9/1 -> Divide1/2
  Product8/1 -> Product7/1
  Add2/1 -> Add5/1
  Add5/1 -> Cn/1
  Product7/1 -> Add5/2
  Beta/1 -> Gain3/1
  del_r/1 -> Gain1/1
  del_a/1 -> Gain2/1
  V/1 -> Gain/1
  P_s/1 -> Gain4/1
  Alpha/1 -> Trigonometric Function/1
  CY/1 -> Product6/2
  Gain2/1 -> Add3/2
  R_s/1 -> Gain5/1

== system UAS_Model_library/External Forces/Aerodynamics/Wind-axes Velocitie/Rates in Wind Axes ==
  note: Rates in Wind Axes
  Alpha_Beta_V : Inport
  PQR : Inport  Port=2
  Alpha : Selector  InputPortWidth=3  IndexOptions=Index vector (dialog)  Indices=[1]  OutputSizes=1
  Beta_Ref : Constant  Value=0
  Direction Cosine Matrix Body to Wind : aerolibtransform2/Direction Cosine Matrix Body to Wind
      settings: SourceProductName=Aerospace Blockset  SourceProductBaseCode=AE
  Mux : Mux  Inputs=2
  transform to body axes : Product  Inputs=**  Multiplication=Matrix(*)  SaturateOnIntegerOverflow=on  InputSameDT=on  OutDataTypeStr=Inherit: Same as first input
  PQR_s : Outport
  wires:
  Alpha_Beta_V/1 -> Alpha/1
  Alpha/1 -> Mux/1
  Direction Cosine Matrix Body to Wind/1 -> transform to body axes/1  "cB_W"
  PQR/1 -> transform to body axes/2
  transform to body axes/1 -> PQR_s/1
  Mux/1 -> Direction Cosine Matrix Body to Wind/1
  Beta_Ref/1 -> Mux/2

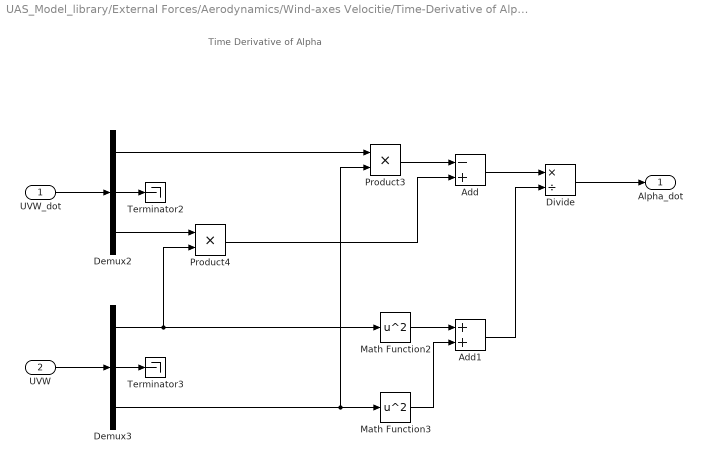
== system UAS_Model_library/External Forces/Aerodynamics/Wind-axes Velocitie/Time-Derivative of Alpha ==
  note: Time Derivative of Alpha
  UVW_dot : Inport
  UVW : Inport  Port=2
  Add : Sum  Inputs=-+
  Add1 : Sum
  Demux2 : Demux  Outputs=3
  Demux3 : Demux  Outputs=3
  Divide : Product  Inputs=*/
  Math Function2 : Math  Operator=square  SaturateOnIntegerOverflow=on
  Math Function3 : Math  Operator=square  SaturateOnIntegerOverflow=on
  Product3 : Product
  Product4 : Product
  Terminator2 : Terminator
  Terminator3 : Terminator
  Alpha_dot : Outport
  wires:
  UVW_dot/1 -> Demux2/1
  Demux2/2 -> Terminator2/1
  Demux2/1 -> Product3/1
  UVW/1 -> Demux3/1
  Demux3/2 -> Terminator3/1
  Demux3/3 -> Math Function3/1, Product3/2
  Demux2/3 -> Product4/1
  Demux3/1 -> Math Function2/1, Product4/2
  Product4/1 -> Add/2
  Product3/1 -> Add/1
  Add/1 -> Divide/1
  Math Function2/1 -> Add1/1
  Math Function3/1 -> Add1/2
  Add1/1 -> Divide/2
  Divide/1 -> Alpha_dot/1
